simulink model "projekatSimulink"  (R2023b)
settings: Solver=FixedStepAuto  StartTime=0.0  StopTime=1000.0  FixedStep=0.1  RelTol=1e-3
libraries: fuzblock x5
settings Model: Creator=Korisnik  LastModifiedBy=Korisnik

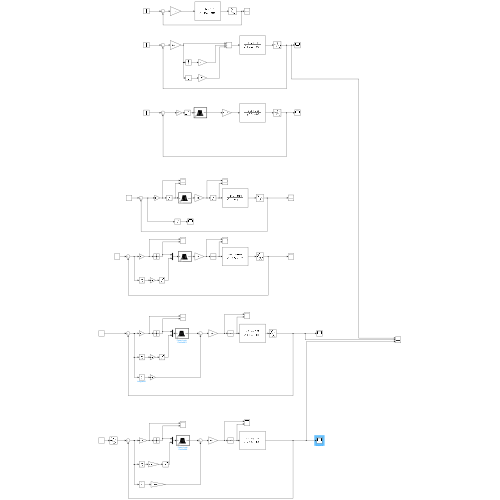
[thumbnail: Simulink's stored preview of the top-level diagram]
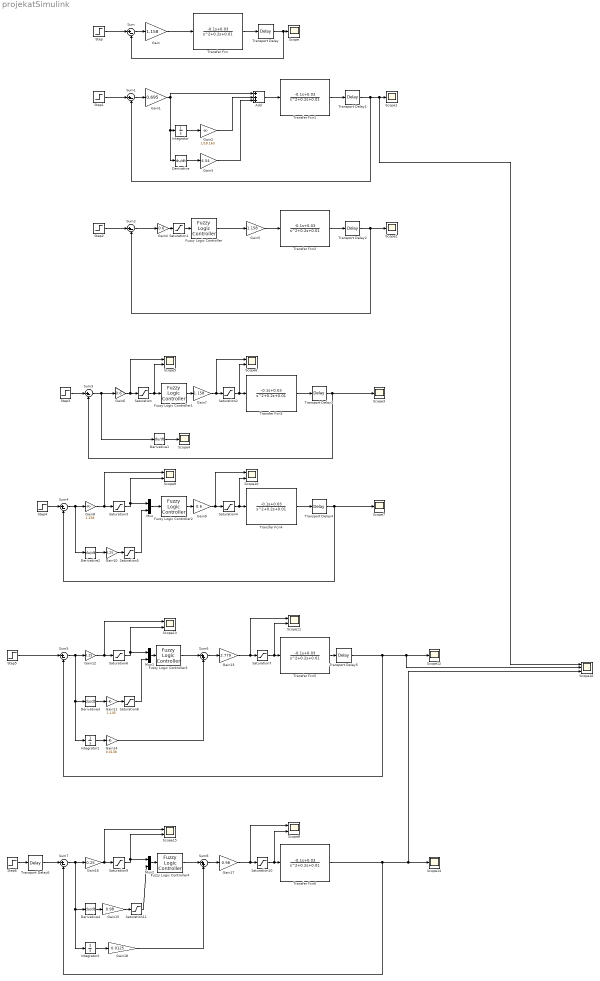
== system projekatSimulink ==
  Add : Sum  Inputs=+++
  Derivative{,1..4} (5 alike) : Derivative
  Fuzzy Logic Controller : fuzblock/Fuzzy Logic  Controller  FIS='FuzzyP'  OutputSampleNumber=101  DataType=double  FuzzifiedInputs=off  RuleFiringStrengths=off  RuleOutputs=off  AggregatedOutputs=off  SimulateUsing=Interpreted execution  OutOfRangeInputValueMessage=warning  NoRuleFiredMessage=warning  EmptyOutputFuzzySetMessage=warning
  Fuzzy Logic Controller1 : fuzblock/Fuzzy Logic  Controller  FIS='FuzzyP'  OutputSampleNumber=101  DataType=double  FuzzifiedInputs=off  RuleFiringStrengths=off  RuleOutputs=off  AggregatedOutputs=off  SimulateUsing=Interpreted execution  OutOfRangeInputValueMessage=warning  NoRuleFiredMessage=warning  EmptyOutputFuzzySetMessage=warning
  Fuzzy Logic Controller2 : fuzblock/Fuzzy Logic  Controller  FIS='FuzzyPD'  OutputSampleNumber=101  DataType=double  FuzzifiedInputs=off  RuleFiringStrengths=off  RuleOutputs=off  AggregatedOutputs=off  SimulateUsing=Interpreted execution  OutOfRangeInputValueMessage=warning  NoRuleFiredMessage=warning  EmptyOutputFuzzySetMessage=warning
  Fuzzy Logic Controller3 : fuzblock/Fuzzy Logic  Controller  FIS='FuzzyPD'  OutputSampleNumber=101  DataType=double  FuzzifiedInputs=off  RuleFiringStrengths=off  RuleOutputs=off  AggregatedOutputs=off  SimulateUsing=Interpreted execution  OutOfRangeInputValueMessage=warning  NoRuleFiredMessage=warning  EmptyOutputFuzzySetMessage=warning
  Fuzzy Logic Controller4 : fuzblock/Fuzzy Logic  Controller  FIS='FuzzyPDnonlinear'  OutputSampleNumber=101  DataType=double  FuzzifiedInputs=off  RuleFiringStrengths=off  RuleOutputs=off  AggregatedOutputs=off  SimulateUsing=Interpreted execution  OutOfRangeInputValueMessage=warning  NoRuleFiredMessage=warning  EmptyOutputFuzzySetMessage=warning
  Gain{,5,7..8} (4 alike) : Gain  Gain=1.158
  Gain1 : Gain  Gain=0.695
  Gain10 : Gain  Gain=5.25
  Gain11 : Gain  Gain=1.135
  Gain12 : Gain  Gain=0.25
  Gain13 : Gain  Gain=2.779
  Gain14 : Gain  Gain=0.0138
  Gain15 : Gain  Gain=0.98
  Gain16 : Gain  Gain=0.25
  Gain17 : Gain  Gain=0.98
  Gain18 : Gain  Gain=0.0125
  Gain2 : Gain  Gain=1/18.163
  Gain3 : Gain  Gain=4.54
  Gain4 : Gain  Gain=0.6
  Gain6 : Gain  Gain=0.6
  Gain9 : Gain  Gain=0.6
  Integrator : Integrator
  Integrator1 : Integrator
  Integrator2 : Integrator
  Mux : Mux  Inputs=2
  Mux1 : Mux  Inputs=2
  Mux2 : Mux  Inputs=2
  Saturation{,1,3,6,9,11} (6 alike) : Saturate  UpperLimit=1  LowerLimit=-1
  Saturation{2,4,7,10} (4 alike) : Saturate  UpperLimit=1.2  LowerLimit=-1.2
  Saturation5 : Saturate  UpperLimit=2  LowerLimit=-2
  Saturation8 : Saturate  UpperLimit=2  LowerLimit=-2
  Scope{,1..4,7,12,14} (8 alike) : Scope
  Scope{5..6,8..11,13,15} (8 alike) : Scope  NumInputPorts=2
  Scope16 : Scope  NumInputPorts=3
  Step{,1..6} (7 alike) : Step  Time=500  Before=-2  After=2  SampleTime=0
  Sum{,1..5,7} (7 alike) : Sum  Inputs=|+-
  Sum6 : Sum  Inputs=|++
  Sum8 : Sum  Inputs=|++
  Transfer Fcn{,1..6} (7 alike) : TransferFcn  Numerator=[-0.1 0.03]  Denominator=[1 0.2 0.01]
  Transport Delay{,1..6} (7 alike) : TransportDelay  DelayTime=3
  wires:
  Gain/1 -> Transfer Fcn/1
  Step/1 -> Sum/1
  Sum/1 -> Gain/1
  Transfer Fcn/1 -> Transport Delay/1
  Transport Delay/1 -> Sum/2, Scope/1
  Transfer Fcn1/1 -> Transport Delay1/1
  Sum1/1 -> Gain1/1
  Step1/1 -> Sum1/1
  Gain1/1 -> Add/1, Integrator/1, Derivative/1
  Integrator/1 -> Gain2/1
  Derivative/1 -> Gain3/1
  Gain2/1 -> Add/2
  Gain3/1 -> Add/3
  Add/1 -> Transfer Fcn1/1
  Step2/1 -> Sum2/1
  Sum2/1 -> Gain4/1
  Gain5/1 -> Transfer Fcn2/1
  Transfer Fcn2/1 -> Transport Delay2/1
  Transport Delay2/1 -> Sum2/2, Scope2/1
  Fuzzy Logic Controller/1 -> Gain5/1
  Step3/1 -> Sum3/1
  Fuzzy Logic Controller1/1 -> Gain7/1
  Sum3/1 -> Gain6/1, Derivative1/1
  Transfer Fcn3/1 -> Transport Delay3/1
  Derivative1/1 -> Scope4/1
  Gain6/1 -> Saturation/1, Scope5/1
  Gain4/1 -> Saturation1/1
  Saturation1/1 -> Fuzzy Logic Controller/1
  Saturation/1 -> Scope5/2, Fuzzy Logic Controller1/1
  Gain7/1 -> Scope6/1, Saturation2/1
  Saturation2/1 -> Scope6/2, Transfer Fcn3/1
  Gain9/1 -> Saturation4/1, Scope10/1
  Fuzzy Logic Controller2/1 -> Gain9/1
  Saturation3/1 -> Mux/1, Scope9/2
  Step4/1 -> Sum4/1
  Sum4/1 -> Gain8/1, Derivative2/1
  Transfer Fcn4/1 -> Transport Delay4/1
  Saturation4/1 -> Scope10/2, Transfer Fcn4/1
  Gain8/1 -> Saturation3/1, Scope9/1
  Mux/1 -> Fuzzy Logic Controller2/1
  Derivative2/1 -> Gain10/1
  Gain10/1 -> Saturation5/1
  Saturation5/1 -> Mux/2
  Transport Delay3/1 -> Scope3/1, Sum3/2
  Saturation7/1 -> Scope11/2, Transfer Fcn5/1
  Gain12/1 -> Saturation6/1, Scope13/1
  Mux1/1 -> Fuzzy Logic Controller3/1
  Gain11/1 -> Saturation8/1
  Saturation8/1 -> Mux1/2
  Derivative3/1 -> Gain11/1
  Saturation6/1 -> Mux1/1, Scope13/2
  Step5/1 -> Sum5/1
  Sum5/1 -> Gain12/1, Integrator1/1, Derivative3/1
  Transport Delay5/1 -> Scope12/1, Scope16/2, Sum5/2
  Transfer Fcn5/1 -> Transport Delay5/1
  Gain13/1 -> Saturation7/1, Scope11/1
  Transport Delay4/1 -> Scope7/1, Sum4/2
  Integrator1/1 -> Gain14/1
  Sum6/1 -> Gain13/1
  Gain14/1 -> Sum6/2
  Fuzzy Logic Controller3/1 -> Sum6/1
  Integrator2/1 -> Gain18/1
  Gain18/1 -> Sum8/2
  Sum8/1 -> Gain17/1
  Gain15/1 -> Saturation11/1
  Transfer Fcn6/1 -> Scope16/3, Scope14/1, Sum7/2
  Saturation11/1 -> Mux2/2
  Mux2/1 -> Fuzzy Logic Controller4/1
  Gain16/1 -> Saturation9/1, Scope15/1
  Derivative4/1 -> Gain15/1
  Fuzzy Logic Controller4/1 -> Sum8/1
  Gain17/1 -> Saturation10/1, Scope8/1
  Saturation10/1 -> Scope8/2, Transfer Fcn6/1
  Saturation9/1 -> Mux2/1, Scope15/2
  Sum7/1 -> Gain16/1, Integrator2/1, Derivative4/1
  Transport Delay1/1 -> Sum1/2, Scope16/1, Scope1/1
  Step6/1 -> Transport Delay6/1
  Transport Delay6/1 -> Sum7/1
